simulink model "PWM Step Test"  (R2025a)
settings: Solver=FixedStepDiscrete  StartTime=0.0  StopTime=Inf  FixedStep=0.01  RelTol=1e-3  EnableMultiTasking=on
model workspace (MAT data in the model file):
  R_motor = 9.6
  encoderDt = 0.02
  k_motor = 0.432432432432
  r = 0.0065
undefined symbols (not defined in the file or in its folder): DiscIntNeverNeededParam
libraries: arduinolib x5, dspstat3 x2, simulink x1, slpidlib x1, arduinosensorlib x1
settings Model: SimulationMode=external  SILPILModeSetting=veronly  ExtModeTrigDuration=2  Creator=Hudso  LastModifiedBy=Hudso
settings SolverCC: AutoInsertRateTranBlk=on
settings OptimizationCC: EnhancedBackFolding=on  PassReuseOutputArgsAs=Individual arguments  ZeroExternalMemoryAtStartup=off  ZeroInternalMemoryAtStartup=off  MaxStackSize=64  OptimizeBlockOrder=speed  DifferentSizesBufferReuse=on  OptimizationCustomize=off  EfficientTunableParamExpr=on
settings DebuggingCC: ParameterTunabilityLossMsg=error
settings HardwareCC: ProdBitPerInt=16.0  ProdBitPerPointer=16.0  ProdBitPerSizeT=16.0  ProdBitPerPtrDiffT=16.0  ProdLargestAtomicFloat=None  ProdWordSize=8.0  ProdHWDeviceType=Atmel->AVR  UseEmbeddedCoderFeatures=off
settings SFSimCC: MATLABDynamicMemAlloc=off
settings RTWCC: SystemTargetFile=ert.tlc  HardwareBoard=Arduino Uno  TemplateMakefile=ert_default_tmf  Toolchain=Arduino AVR  BuildConfiguration=Faster Runs  Description=Embedded Coder
settings CodeAppCC: ForceParamTrailComments=on  IgnoreCustomStorageClasses=off  OperatorAnnotations=on  SimulinkDataObjDesc=on  SFDataObjDesc=on  InsertBlockDesc=on
settings ERTTargetCC: ExtModeTransport=3.0  ExtModeAutomaticAllocSize=off  ExtModeStaticAllocSize=250.0  InlinedParameterPlacement=Hierarchical  SupportContinuousTime=on  SupportNonInlinedSFcns=on  SupportVariableSizeSignals=on

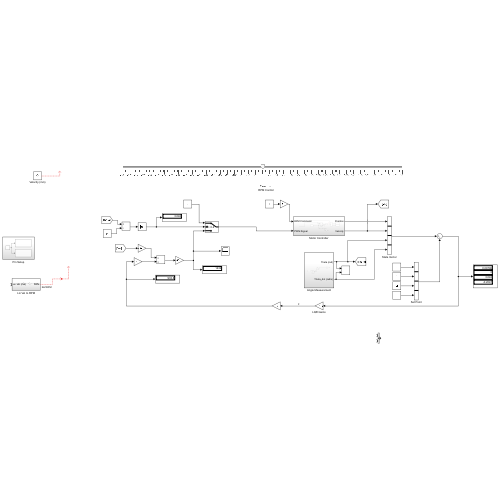
[thumbnail: Simulink's stored preview of the top-level diagram]
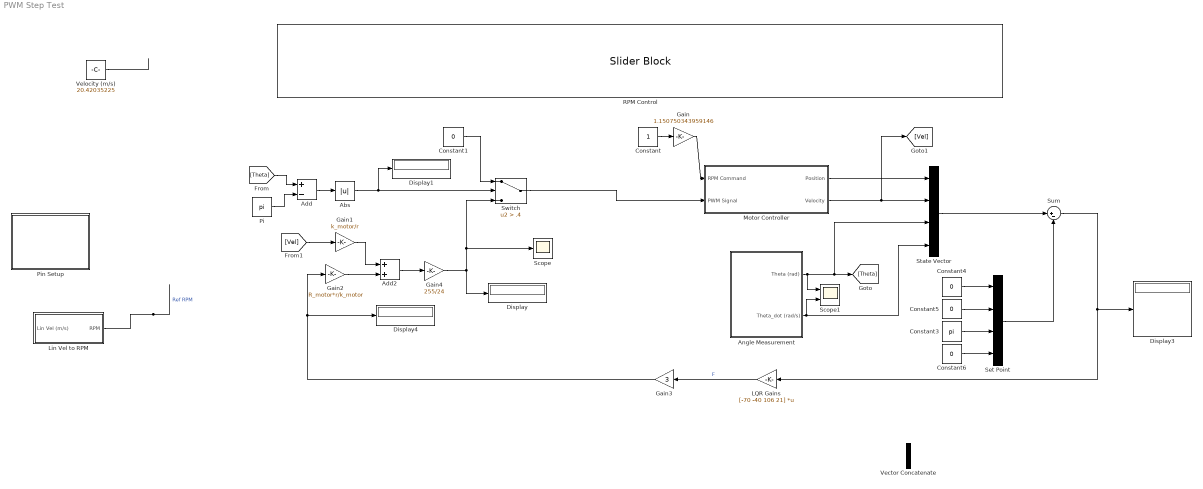
== system PWM Step Test ==
  Abs : Abs  SaturateOnIntegerOverflow=off
  Add : Sum  Inputs=+-
  Add2 : Sum
  Angle Measurement : Subsystem
  Constant : Constant
  Constant{1,4..6} (4 alike) : Constant  Value=0
  Constant3 : Constant  Value=pi
  Display{,1,3..4} (4 alike) : Display
  Gain : Gain  Gain=1.150750343959146
  Gain1 : Gain  Gain=k_motor/r
  Gain2 : Gain  Gain=R_motor*r/k_motor
  Gain3 : Gain  Gain=3
  Gain4 : Gain  Gain=255/24
  LQR Gains : Gain  Gain=[-70 -40 106 21]  Multiplication=Matrix(K*u)
  Lin Vel to RPM : Subsystem
  Motor Controller : Subsystem
  Pi : Constant  Value=pi  OutDataTypeStr=Inherit: Inherit via back propagation
  Pin Setup : Subsystem
  RPM Control : SliderBlock  LabelPosition=Bottom  ScaleMin=-500  ScaleMax=500
  Scope : Scope
      settings: ActiveDisplayYMinimum=-610.5649621770242  ActiveDisplayYMaximum=-410.56496217702426
  Scope1 : Scope  NumInputPorts=2
      settings: ActiveDisplayYMinimum=-15.589420003091735  ActiveDisplayYMaximum=15.099016698040856  DataLoggingVariableName=ScopeData2
  Set Point : Concatenate  NumInputs=4
  State Vector : Concatenate  NumInputs=4
  Sum : Sum  Inputs=|+-
  Switch : Switch  Criteria=u2 > Threshold  Threshold=.4  SaturateOnIntegerOverflow=off  InputSameDT=off
  Vector Concatenate : Concatenate
  Velocity (m/s) : Constant  Value=20.42035225
  wires:
  Velocity (m/s)/1 -> ?
  Angle Measurement/1(Theta (rad)) -> State Vector/3, [Theta], Scope1/1
  Motor Controller/1(Position) -> State Vector/1
  Motor Controller/2(Velocity) -> [Vel], State Vector/2
  Angle Measurement/2(Theta_dot (rad/s)) -> State Vector/4, Scope1/2
  Lin Vel to RPM/1(RPM) -> ?  "Ref RPM"
  Gain/1 -> Motor Controller/1(RPM Command)
  Constant/1 -> Gain/1
  Constant1/1 -> Switch/1
  Switch/1 -> Motor Controller/2(PWM Signal)
  [Theta] -> Add/1
  Pi/1 -> Add/2
  Add/1 -> Abs/1
  Abs/1 -> Display1/1, Switch/2
  LQR Gains/1 -> Gain3/1  "F"
  Gain1/1 -> Add2/1
  [Vel] -> Gain1/1
  Add2/1 -> Gain4/1
  Gain3/1 -> Display4/1, Gain2/1
  Gain2/1 -> Add2/2
  Gain4/1 -> Scope/1, Switch/3, Display/1
  Constant3/1 -> Set Point/3
  Constant4/1 -> Set Point/1
  Constant5/1 -> Set Point/2
  Constant6/1 -> Set Point/4
  State Vector/1 -> Sum/1
  Sum/1 -> Display3/1, LQR Gains/1
  Set Point/1 -> Sum/2

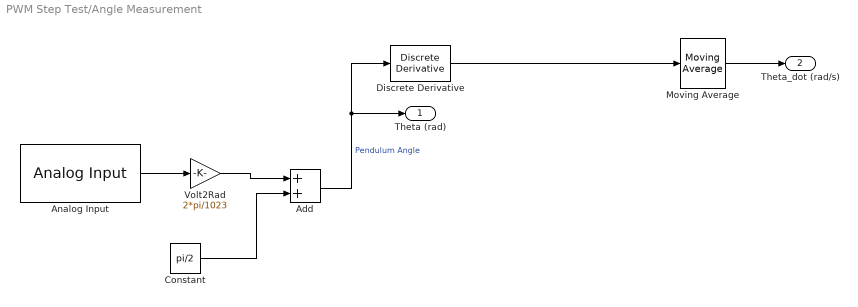
== system PWM Step Test/Angle Measurement ==
  Add : Sum
  Analog Input : arduinolib/Analog Input  pinNumber=0  ReadResultsOnly=off  ConversionTriggerSource=Software  ExternalTriggerType=uint32( 0 )  OutputDataType=uint16  EnableConversionCompleteNotify=off  EnableOuputStatus=off  SampleTime=-1  blockPlatform=arduino
  Constant : Constant  Value=pi/2
  Discrete Derivative : simulink/Discrete/Discrete Derivative  gainval=1.0  ICPrevScaledInput=0.0  OutMin=[]  OutMax=[]  OutDataType=fixdt(1, 16)  OutScaling=2^-10  DoSatur=off
  Moving Average : dspstat3/Moving Average  Method=Sliding window  ForgettingFactorPort=off  SpecifyWindowLength=on  WindowLength=3  OverlapLength=2  AllowArbitraryInputLength=off  ForgettingFactor=0.95  SimulateUsing=Interpreted execution
  Volt2Rad : Gain  Gain=2*pi/1023
  Theta (rad) : Outport
  Theta_dot (rad/s) : Outport  Port=2
  wires:
  Volt2Rad/1 -> Add/1
  Analog Input/1 -> Volt2Rad/1
  Add/1 -> Discrete Derivative/1, Theta (rad)/1  "Pendulum Angle"
  Discrete Derivative/1 -> Moving Average/1
  Moving Average/1 -> Theta_dot (rad/s)/1
  Constant/1 -> Add/2

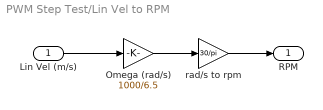
== system PWM Step Test/Lin Vel to RPM ==
  Lin Vel (m/s) : Inport
  Omega (rad/s) : Gain  Gain=1000/6.5
  rad/s to rpm : Gain  Gain=30/pi
  RPM : Outport
  wires:
  Lin Vel (m/s)/1 -> Omega (rad/s)/1
  Omega (rad/s)/1 -> rad/s to rpm/1
  rad/s to rpm/1 -> RPM/1

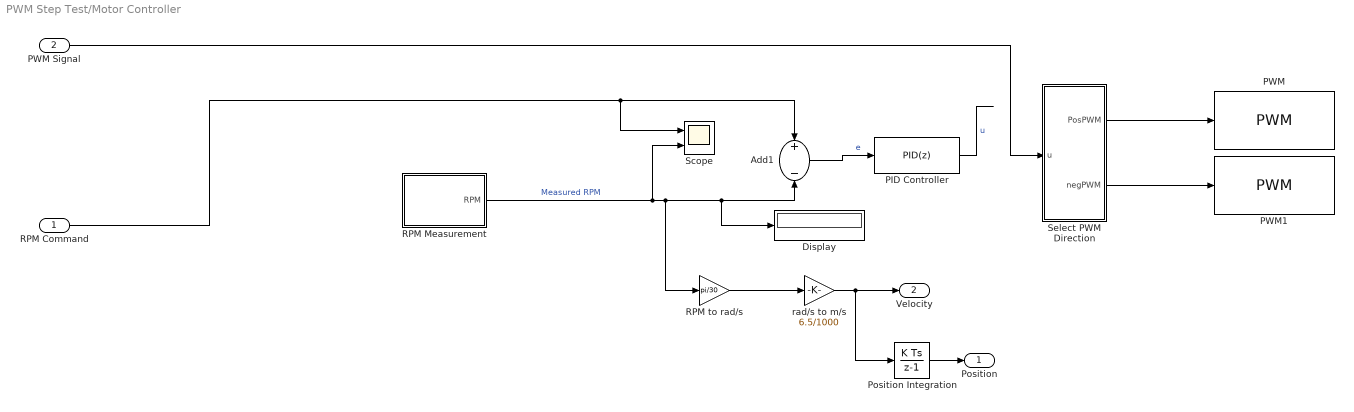
== system PWM Step Test/Motor Controller ==
  RPM Command : Inport
  PWM Signal : Inport  Port=2
  Add1 : Sum  Inputs=+-
  Display : Display
  PID Controller : slpidlib/PID Controller  Controller=PID  Form=Parallel  TimeDomain=Discrete-time  UseExternalTs=off  SampleTime=encoderDt  IntegratorMethod=Forward Euler  FilterMethod=Forward Euler  ControllerParametersSource=internal  P=.43  I=6  UseKiTs=off  D=0.02  UseExternalDerivativeSource=off  N=2  UseFilter=on  TunerSelectOption=Transfer Function Based (PID Tuner App)  InitialConditionSource=internal  InitialConditionForIntegrator=0  InitialConditionForFilter=0  DifferentiatorICPrevScaledInput=0  ExternalReset=none  TrackingMode=off  Kt=1  LimitOutput=on  SatLimitsSource=internal  UpperSaturationLimit=255  LowerSaturationLimit=-255  LinearizeAsGain=off  AntiWindupMode=back-calculation  Kb=.1  LimitIntegrator=off  UpperIntegratorSaturationLimit=inf  LowerIntegratorSaturationLimit=-inf  POutMin=[]  POutMax=[]  IOutMin=[]  IOutMax=[]  DOutMin=[]  DOutMax=[]  NOutMin=[]  NOutMax=[]  SumOutMin=[]  SumOutMax=[]  SaturationOutMin=[]  SaturationOutMax=[]  PParamMin=[]  PParamMax=[]  IParamMin=[]  IParamMax=[]  DParamMin=[]  DParamMax=[]  NParamMin=[]  NParamMax=[]  KbParamMin=[]  KbParamMax=[]  KtParamMin=[]  KtParamMax=[]  KbOutMin=[]  KbOutMax=[]  KtOutMin=[]  KtOutMax=[]  IntegratorOutMin=[]  IntegratorOutMax=[]  FilterOutMin=[]  FilterOutMax=[]  SumI1OutMin=[]  SumI1OutMax=[]  SumI2OutMin=[]  SumI2OutMax=[]  SumI3OutMin=[]  SumI3OutMax=[]  SumI4OutMin=[]  SumI4OutMax=[]  SumDOutMin=[]  SumDOutMax=[]  DifferentiatorOutMin=[]  DifferentiatorOutMax=[]  FilterDiffOutCoefMin=[]  FilterDiffOutCoefMax=[]  ReciprocalOutMin=[]  ReciprocalOutMax=[]  SumDenOutMin=[]  SumDenOutMax=[]  SumNumOutMin=[]  SumNumOutMax=[]  DivideOutMin=[]  DivideOutMax=[]  UdiffTsProdOutMin=[]  UdiffTsProdOutMax=[]  NTsProdOutMin=[]  NTsProdOutMax=[]  UintegralTsProdOutMin=[]  UintegralTsProdOutMax=[]  UngainTsProdOutMin=[]  UngainTsProdOutMax=[]  ClampingZeroOutDataTypeStr=Inherit: Inherit via back propagation  ClampingZeroOutMin=[]  ClampingZeroOutMax=[]  FilterDenConstantOutDataTypeStr=Inherit: Inherit via back propagation  FilterDenConstantOutMin=[]  FilterDenConstantOutMax=[]  PCopyOutDataTypeStr=Inherit: Inherit via back propagation  PCopyOutMin=[]  PCopyOutMax=[]  NCopyOutDataTypeStr=Inherit: Inherit via back propagation  NCopyOutMin=[]  NCopyOutMax=[]  IntegratorContinuousStateAttributes=''  IntegratorStateMustResolveToSignalObject=off  IntegratorRTWStateStorageClass=Auto  FilterContinuousStateAttributes=''  FilterStateMustResolveToSignalObject=off  FilterRTWStateStorageClass=Auto  ParallelPVariant=InternalParameters  IdealPVariant=Disabled  IVariant=InternalParameters  DVariant=InternalParameters  IntegratorVariant=Discrete  SatVariant=Enabled  AWVariant=BackCalculation  PCopyVariant=Disabled  TRVariant=Disabled  FdbkBlocksVariant=Forward  IdealPFdbkVariant=Disabled  SatFdbkVariant=Disabled  DerivativeFilterVariant=ForwardEulerFilter  NVariant=InternalParameters  NCopyVariant=Disabled  FilterICVariant=InternalICsFilter  IntegratorICVariant=InternalICs  ExternalResetVariant=Disabled  TRSumVariant=Passthrough  SumFdbkVariant=Disabled  SumVariant=Sum_PID  TsampFilterVariant=InternalTs  TsampNgainVariant=Passthrough  TsampIntegralVariant=Disabled_SignalSpec  ExternalSaturationOutDataTypeStr=Inherit: Same as second input  DerivativeSourceVariant=ErrorSignal  PreIntVariant=InternalPreInt
  PWM : arduinolib/PWM  pinNumber=5  frequencyType=Default  desiredFrequency=490.2  achievableFrequency=490.2
  PWM1 : arduinolib/PWM  pinNumber=6  frequencyType=Default  desiredFrequency=490.2  achievableFrequency=490.2
  Position Integration : DiscreteIntegrator  SampleTime=encoderDt  ICPrevOutput=DiscIntNeverNeededParam  ICPrevScaledInput=DiscIntNeverNeededParam
  RPM Measurement : Subsystem
  RPM to rad/s : Gain  Gain=pi/30
  Scope : Scope  NumInputPorts=2
      settings: ActiveDisplayYMinimum=-1040.4893566754752  ActiveDisplayYMaximum=1748.3640890647034
  Select PWM Direction : MATLAB Function  TreatAsAtomicUnit=on
  rad/s to m/s : Gain  Gain=6.5/1000
  Position : Outport
  Velocity : Outport  Port=2
  wires:
  RPM to rad/s/1 -> rad/s to m/s/1
  Add1/1 -> PID Controller/1  "e"
  Select PWM Direction/2(negPWM) -> PWM1/1
  RPM Measurement/1(RPM) -> Scope/2, RPM to rad/s/1, Display/1, Add1/2  "Measured RPM"
  Position Integration/1 -> Position/1
  RPM Command/1 -> Add1/1, Scope/1
  PID Controller/1 -> ?  "u"
  Select PWM Direction/1(PosPWM) -> PWM/1
  rad/s to m/s/1 -> Position Integration/1, Velocity/1
  PWM Signal/1 -> Select PWM Direction/1(u)

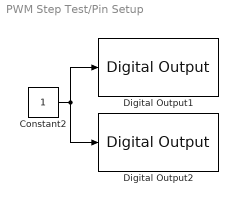
== system PWM Step Test/Pin Setup ==
  Constant2 : Constant
  Digital Output1 : arduinolib/Digital Output  pinNumber=7  Direction=output  blockPlatform=arduino
  Digital Output2 : arduinolib/Digital Output  pinNumber=8  Direction=output  blockPlatform=arduino
  wires:
  Constant2/1 -> Digital Output1/1, Digital Output2/1

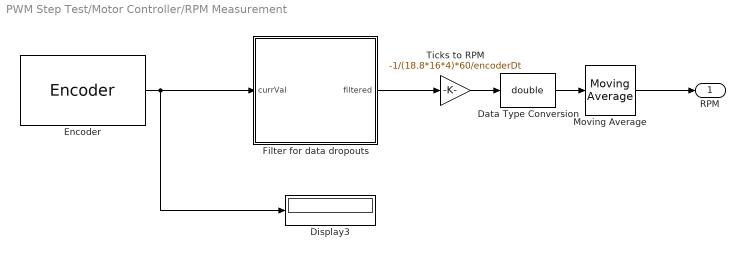
== system PWM Step Test/Motor Controller/RPM Measurement ==
  Data Type Conversion : DataTypeConversion  OutDataTypeStr=double  SaturateOnIntegerOverflow=off  RndMeth=Floor
  Display3 : Display
  Encoder : arduinosensorlib/Encoder  InputA=2  InputB=3  Mode=Reset at each Sample time  SampleTime=encoderDt
  Filter for data dropouts : MATLAB Function  TreatAsAtomicUnit=on
  Moving Average : dspstat3/Moving Average  Method=Sliding window  ForgettingFactorPort=off  SpecifyWindowLength=on  WindowLength=4  OverlapLength=3  AllowArbitraryInputLength=off  ForgettingFactor=0.9  SimulateUsing=Interpreted execution
  Ticks to RPM : Gain  Gain=-1/(18.8*16*4)*60/encoderDt
  RPM : Outport
  wires:
  Filter for data dropouts/1(filtered) -> Ticks to RPM/1
  Encoder/1 -> Display3/1, Filter for data dropouts/1(currVal)
  Ticks to RPM/1 -> Data Type Conversion/1
  Data Type Conversion/1 -> Moving Average/1
  Moving Average/1 -> RPM/1

== matlab function PWM Step Test/Motor Controller/RPM Measurement/Filter for data dropouts ==
  data: currVal input; filtered output
function filtered = filterEncoder(currVal)
%#codegen

persistent prevVal

% Initialize on first call
if isempty(prevVal)
    prevVal = currVal;
end

% Dropout detection
threshold = 200;  % Adjust based on your system

if abs(currVal - prevVal) > threshold
    % Bad reading: keep previous good value
    filtered = prevVal;
else
    % Good reading: update and pass through
    filtered = currVal;
    prevVal = currVal;
end

== matlab function PWM Step Test/Motor Controller/Select PWM Direction ==
  data: u input; PosPWM output; negPWM output
function [PosPWM, negPWM] = PWMDir(u)
    if u > 0
        PosPWM = u;
        negPWM = 0;
    else
        negPWM = -u;
        PosPWM = 0;
    end
end
